simulink model "input_output_feedback"  (R2024b)
settings: Solver=FixedStepAuto  StartTime=0.0  StopTime=Tf  FixedStep=Tn  RelTol=1e-3
undefined symbols (not defined in the file or in its folder): k1, k2
libraries: robotmobilelib x1
settings Model: Creator=fiore  LastModifiedBy=fiore

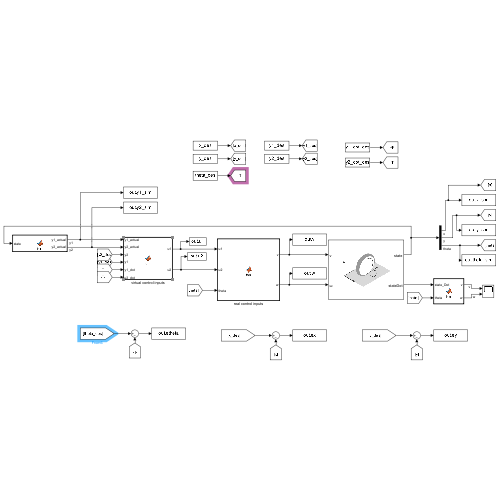
[thumbnail: Simulink's stored preview of the top-level diagram]
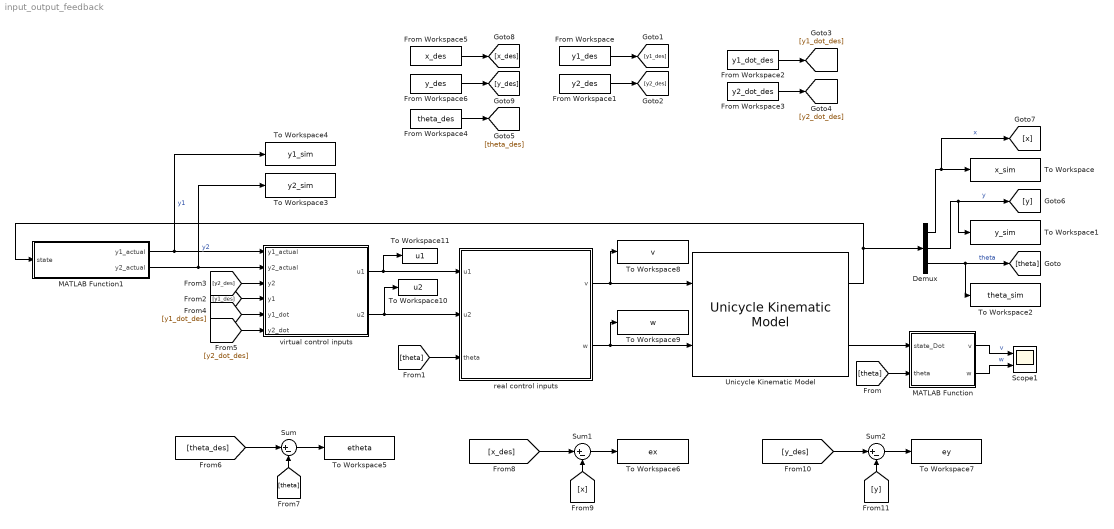
== system input_output_feedback ==
  Demux : Demux  Outputs=3
  From Workspace : FromWorkspace  VariableName=y1_des
  From Workspace1 : FromWorkspace  VariableName=y2_des
  From Workspace2 : FromWorkspace  VariableName=y1_dot_des
  From Workspace3 : FromWorkspace  VariableName=y2_dot_des
  From Workspace4 : FromWorkspace  VariableName=theta_des
  From Workspace5 : FromWorkspace  VariableName=x_des
  From Workspace6 : FromWorkspace  VariableName=y_des
  MATLAB Function : MATLAB Function  TreatAsAtomicUnit=on
  MATLAB Function1 : MATLAB Function  TreatAsAtomicUnit=on
  Scope1 : Scope  NumInputPorts=2
  Sum : Sum  Inputs=|+-
  Sum1 : Sum  Inputs=|+-
  Sum2 : Sum  Inputs=|+-
  To Workspace : ToWorkspace  VariableName=x_sim  SaveFormat=Timeseries  SampleTime=-1
  To Workspace1 : ToWorkspace  VariableName=y_sim  SaveFormat=Timeseries  SampleTime=-1
  To Workspace10 : ToWorkspace  VariableName=u2  SaveFormat=Timeseries  SampleTime=-1
  To Workspace11 : ToWorkspace  VariableName=u1  SaveFormat=Timeseries  SampleTime=-1
  To Workspace2 : ToWorkspace  VariableName=theta_sim  SaveFormat=Timeseries  SampleTime=-1
  To Workspace3 : ToWorkspace  VariableName=y2_sim  SaveFormat=Timeseries  SampleTime=-1
  To Workspace4 : ToWorkspace  VariableName=y1_sim  SaveFormat=Timeseries  SampleTime=-1
  To Workspace5 : ToWorkspace  VariableName=etheta  SaveFormat=Timeseries  SampleTime=-1
  To Workspace6 : ToWorkspace  VariableName=ex  SaveFormat=Timeseries  SampleTime=-1
  To Workspace7 : ToWorkspace  VariableName=ey  SaveFormat=Timeseries  SampleTime=-1
  To Workspace8 : ToWorkspace  VariableName=v  SaveFormat=Timeseries  SampleTime=-1
  To Workspace9 : ToWorkspace  VariableName=w  SaveFormat=Timeseries  SampleTime=-1
  Unicycle Kinematic Model : robotmobilelib/Unicycle Kinematic Model  VehicleInputs=Vehicle Speed & Heading Angular Velocity  WheelRadius=0.05  WheelSpeedRange=[-Inf Inf]  InitialState=qi  SimulateUsing=Interpreted execution
  real control inputs : MATLAB Function  TreatAsAtomicUnit=on
  virtual control inputs : MATLAB Function  TreatAsAtomicUnit=on
  wires:
  virtual control inputs/1(u1) -> To Workspace11/1, real control inputs/1(u1)
  virtual control inputs/2(u2) -> To Workspace10/1, real control inputs/2(u2)
  real control inputs/1(v) -> To Workspace8/1, Unicycle Kinematic Model/1
  real control inputs/2(w) -> To Workspace9/1, Unicycle Kinematic Model/2
  Unicycle Kinematic Model/1 -> Demux/1, MATLAB Function1/1(state)
  Unicycle Kinematic Model/2 -> MATLAB Function/1(state_Dot)
  Demux/3 -> To Workspace2/1, [theta]  "theta"
  [theta] -> MATLAB Function/2(theta)
  [theta] -> real control inputs/3(theta)
  MATLAB Function/1(v) -> Scope1/1  "v"
  MATLAB Function/2(w) -> Scope1/2  "w"
  Demux/1 -> [x], To Workspace/1  "x"
  Demux/2 -> [y], To Workspace1/1  "y"
  From Workspace/1 -> [y1_des]
  From Workspace3/1 -> [y2_dot_des]
  From Workspace2/1 -> [y1_dot_des]
  From Workspace1/1 -> [y2_des]
  [y1_des] -> virtual control inputs/4(y1)
  [y2_des] -> virtual control inputs/3(y2)
  [y1_dot_des] -> virtual control inputs/5(y1_dot)
  [y2_dot_des] -> virtual control inputs/6(y2_dot)
  MATLAB Function1/1(y1_actual) -> To Workspace4/1, virtual control inputs/1(y1_actual)  "y1"
  MATLAB Function1/2(y2_actual) -> To Workspace3/1, virtual control inputs/2(y2_actual)  "y2"
  From Workspace4/1 -> [theta_des]
  [theta_des] -> Sum/1
  [theta] -> Sum/2
  Sum/1 -> To Workspace5/1
  [x_des] -> Sum1/1
  Sum1/1 -> To Workspace6/1
  [x] -> Sum1/2
  [y_des] -> Sum2/1
  [y] -> Sum2/2
  Sum2/1 -> To Workspace7/1
  From Workspace6/1 -> [y_des]
  From Workspace5/1 -> [x_des]

== matlab function input_output_feedback/real control inputs ==
  data: u1 input; v output; u2 input; w output; b parameter; theta input
function [v, w] = fcn(u1, u2, b, theta)
T = [cos(theta), -b*sin(theta);
    sin(theta), b*cos(theta)];
res = inv(T)*[u1; u2];
v = res(1);
w = res(2);
end

== matlab function input_output_feedback/virtual control inputs ==
  data: k1 parameter; k2 parameter; u1 output; u2 output; y1_actual input; y2_actual input; y2 input; y1 input; y1_dot input; y2_dot input
function [u1, u2] = fcn(k1, k2, y1_actual, y2_actual, y2, y1, y1_dot, y2_dot)

u1 = y1_dot + k1*(y1 - y1_actual);
u2 = y2_dot + k2*(y2 - y2_actual);

end

== matlab function input_output_feedback/MATLAB Function1 ==
  data: state input; y1_actual output; y2_actual output; b parameter
function [y1_actual, y2_actual] = fcn(state, b)

x = state(1);
y = state(2);
theta = state(3);

y1_actual = x + b*cos(theta);
y2_actual = y + b*sin(theta);

end

== matlab function input_output_feedback/MATLAB Function ==
  data: state_Dot input; v output; w output; theta input
function [v,w] = fcn(state_Dot,theta)

w = state_Dot(3);
v = state_Dot(1)/cos(theta);

end
